simulink model "StateJacobian"  (R2022b)
settings: Solver=FixedStepAuto  StartTime=0.0  StopTime=10.0  RelTol=1e-3  SampleTimeConstraint=STIndependent
undefined symbols (not defined in the file): NumberSt, NumModules, NumSeries, Ts
settings Model: DataDictionary=Estimators_Dictionary.sldd  Creator=japerez  LastModifiedBy=jgavidia
settings DataIOCC: SaveOutput=off  SaveTime=off
settings DebuggingCC: ParameterPrecisionLossMsg=none

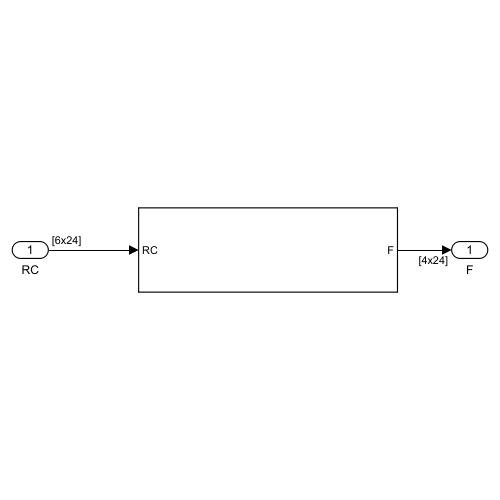
[thumbnail: Simulink's stored preview of the top-level diagram]
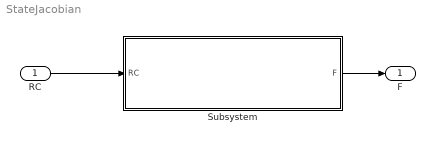
== system StateJacobian ==
  RC : Inport  OutDataTypeStr=single  PortDimensions=[6,NumModules*NumSeries]
  Subsystem : Subsystem
  F : Outport  OutDataTypeStr=single  PortDimensions=[NumberSt,NumModules*NumSeries]
  wires:
  Subsystem/1(F) -> F/1
  RC/1 -> Subsystem/1(RC)

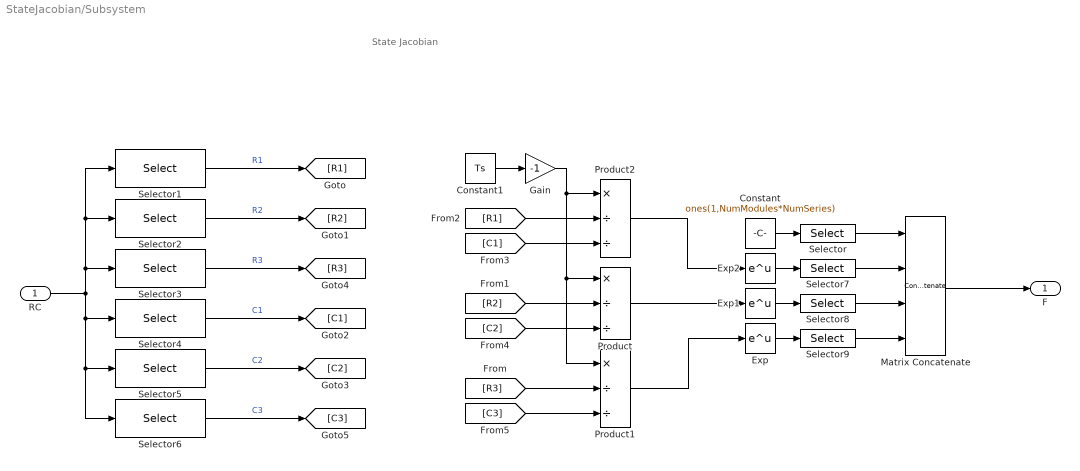
== system StateJacobian/Subsystem ==
  note: State Jacobian
  RC : Inport
  Constant : Constant  Value=ones(1,NumModules*NumSeries)  OutDataTypeStr=single
  Constant1 : Constant  Value=Ts  OutDataTypeStr=single
  Exp : Math
  Exp1 : Math
  Exp2 : Math
  Gain : Gain  Gain=-1
  Matrix Concatenate : Concatenate  NumInputs=4  Mode=Multidimensional array
  Product : Product  Inputs=*//
  Product1 : Product  Inputs=*//
  Product2 : Product  Inputs=*//
  Selector{,7..9} (4 alike) : Selector  NumberOfDimensions=2  InputPortWidth=3  IndexOptions=Select all,Index vector (dialog)  Indices=[1 3],[1:24]  OutputSizes=1,1
  Selector1 : Selector  NumberOfDimensions=2  InputPortWidth=24  IndexOptions=Index vector (dialog),Select all  Indices=1,1  OutputSizes=1,1
  Selector2 : Selector  NumberOfDimensions=2  InputPortWidth=24  IndexOptions=Index vector (dialog),Select all  Indices=2,2  OutputSizes=1,1
  Selector3 : Selector  NumberOfDimensions=2  InputPortWidth=24  IndexOptions=Index vector (dialog),Select all  Indices=3,3  OutputSizes=1,1
  Selector4 : Selector  NumberOfDimensions=2  InputPortWidth=24  IndexOptions=Index vector (dialog),Select all  Indices=4,4  OutputSizes=1,1
  Selector5 : Selector  NumberOfDimensions=2  InputPortWidth=24  IndexOptions=Index vector (dialog),Select all  Indices=5,5  OutputSizes=1,1
  Selector6 : Selector  NumberOfDimensions=2  InputPortWidth=24  IndexOptions=Index vector (dialog),Select all  Indices=6,6  OutputSizes=1,1
  F : Outport
  wires:
  Constant/1 -> Selector/1
  [C3] -> Product1/3
  [R1] -> Product2/2
  Selector3/1 -> [R3]  "R3"
  Selector5/1 -> [C2]  "C2"
  Product1/1 -> Exp/1
  [R2] -> Product/2
  Selector6/1 -> [C3]  "C3"
  Exp/1 -> Selector9/1
  [C2] -> Product/3
  Product2/1 -> Exp2/1
  Constant1/1 -> Gain/1
  Selector4/1 -> [C1]  "C1"
  RC/1 -> Selector1/1, Selector2/1, Selector3/1, Selector5/1, Selector6/1, Selector4/1
  Matrix Concatenate/1 -> F/1
  Exp2/1 -> Selector7/1
  Selector2/1 -> [R2]  "R2"
  Selector1/1 -> [R1]  "R1"
  Gain/1 -> Product2/1, Product/1, Product1/1
  [R3] -> Product1/2
  [C1] -> Product2/3
  Exp1/1 -> Selector8/1
  Product/1 -> Exp1/1
  Selector/1 -> Matrix Concatenate/1
  Selector7/1 -> Matrix Concatenate/2
  Selector8/1 -> Matrix Concatenate/3
  Selector9/1 -> Matrix Concatenate/4
